simulink model "gm_Copy_of_uz_pmsm_model_9ph_21b_all_double"  (R2021b)
settings: Solver=FixedStepAuto  StartTime=0.0  StopTime=0.8  RelTol=1e-3
PreLoadFcn:
  | uz_pmsm_model_9ph_init_parameter
undefined symbols (not defined in the file or in its folder): a, b, c, friction_coefficient, inertia, k_i_d, k_i_q, k_p_d, k_p_q, Kpd, L_d, L_o1, L_o2, L_q, L_x1, L_x2, L_y1, L_y2, L_zero, polepair, psi_pm, R_1, static_friction_torque, Tnd, ts
libraries: hdlsllib x90, hdlmdlgenlib x17, slpidlib x2, simulink x2, spsAlphaBetaZerotodq0Lib x1, pid_lib x1, spsdq0toAlphaBetaZeroLib x1
(part 1 of 3)
settings Model: Creator=ts  LastModifiedBy=ts
settings SolverCC: AlgebraicLoopSolver=TrustRegion  AutoInsertRateTranBlk=on
settings DataIOCC: LimitDataPoints=on  SaveOutput=off  SaveTime=off
settings OptimizationCC: BlockReduction=off  ConditionallyExecuteInputs=off  DefaultParameterBehavior=Inlined  InheritOutputTypeSmallerThanSingle=on  LifeSpan=inf
settings DebuggingCC: AlgebraicLoopMsg=error  InheritedTsInSrcMsg=none  SingleTaskRateTransMsg=error  AllowSymbolicDim=off  StrictBusMsg=ErrorOnBusTreatedAsVector  SFUnexpectedBacktrackingDiag=warning  SFNoUnconditionalDefaultTransitionDiag=warning  SFExecutionAtInitializationDiag=none  SFMachineParentedDataDiag=warning  ArithmeticOperatorsInVariantConditions=warning
settings HardwareCC: ProdBitPerPointer=32  ProdBitPerSizeT=32  ProdBitPerPtrDiffT=32  ProdLargestAtomicFloat=None  ProdIntDivRoundTo=Undefined  ProdEndianess=Unspecified  ProdWordSize=32  ProdHWDeviceType=ASIC/FPGA->ASIC/FPGA  ProdEqTarget=off
settings SFSimCC: SimUseLocalCustomCode=off  CustomCodeUndefinedFunction=UseInterfaceOnly
settings RTWCC: RTWUseLocalCustomCode=off
settings CodeAppCC: StateflowObjectComments=on
settings GRTTargetCC: TargetLangStandard=C89/C90 (ANSI)
settings ConfigComp: CovScope=ReferencedModels  CovMetricSettings=dw  CovSaveCumulativeToWorkspaceVar=on  CovSaveSingleToWorkspaceVar=on  CovExternalEMLEnable=off  CovSFcnEnable=off

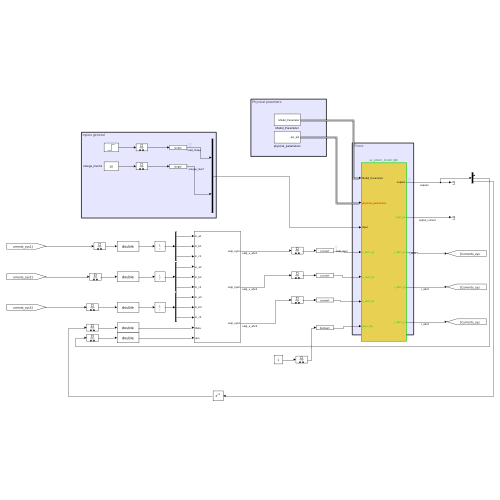
[thumbnail: Simulink's stored preview of the top-level diagram]
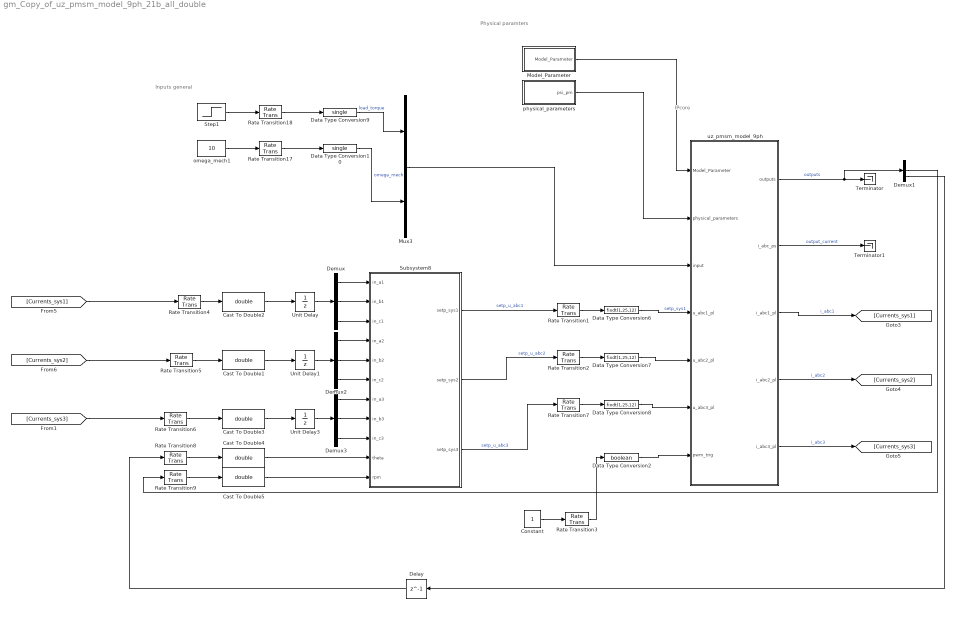
== system gm_Copy_of_uz_pmsm_model_9ph_21b_all_double ==
  note: IPcore
  note: Physical paramters
  note: Inputs general
  Cast To Double{1..5} (5 alike) : DataTypeConversion  OutDataTypeStr=double
  Constant : Constant
  Data Type Conversion10 : DataTypeConversion  OutDataTypeStr=single  RndMeth=Nearest
  Data Type Conversion2 : DataTypeConversion  OutDataTypeStr=boolean  RndMeth=Nearest
  Data Type Conversion6 : DataTypeConversion  OutDataTypeStr=fixdt(1,25,12)  RndMeth=Nearest
  Data Type Conversion7 : DataTypeConversion  OutDataTypeStr=fixdt(1,25,12)  RndMeth=Nearest
  Data Type Conversion8 : DataTypeConversion  OutDataTypeStr=fixdt(1,25,12)  RndMeth=Nearest
  Data Type Conversion9 : DataTypeConversion  OutDataTypeStr=single  RndMeth=Nearest
  Delay : Delay  DelayLength=1
  Demux{,1..3} (4 alike) : Demux  Outputs=3
  Model_Parameter : Subsystem
  Mux3 : Mux  Inputs=2
  Rate Transition{1..3,7,17..18} (6 alike) : RateTransition  OutPortSampleTime=ts
  Rate Transition{4..6,8..9} (5 alike) : RateTransition  OutPortSampleTime=1/10000
  Step1 : Step  Time=0.25  After=20  SampleTime=0
  Subsystem8 : Subsystem
  Terminator : Terminator
  Terminator1 : Terminator
  Unit Delay : UnitDelay  SampleTime=-1  HasFrameUpgradeWarning=on
  Unit Delay1 : UnitDelay  SampleTime=-1  HasFrameUpgradeWarning=on
  Unit Delay3 : UnitDelay  SampleTime=-1  HasFrameUpgradeWarning=on
  omega_mech1 : Constant  Value=10
  physical_parameters : Subsystem
  uz_pmsm_model_9ph : Subsystem  TreatAsAtomicUnit=on
  wires:
  physical_parameters/1(psi_pm) -> uz_pmsm_model_9ph/2(physical_parameters)
  uz_pmsm_model_9ph/1(outputs) -> Demux1/1, Terminator/1  "outputs"
  Model_Parameter/1(Model_Parameter) -> uz_pmsm_model_9ph/1(Model_Parameter)
  omega_mech1/1 -> Rate Transition17/1
  Rate Transition18/1 -> Data Type Conversion9/1
  Step1/1 -> Rate Transition18/1
  Data Type Conversion10/1 -> Mux3/2  "omega_mech"
  Rate Transition17/1 -> Data Type Conversion10/1
  Data Type Conversion9/1 -> Mux3/1  "load_torque"
  Mux3/1 -> uz_pmsm_model_9ph/3(input)
  uz_pmsm_model_9ph/2(i_abc_ps) -> Terminator1/1  "output_current"
  uz_pmsm_model_9ph/3(i_abc1_pl) -> [Currents_sys1]  "i_abc1"
  uz_pmsm_model_9ph/5(i_abc3_pl) -> [Currents_sys3]  "i_abc3"
  uz_pmsm_model_9ph/4(i_abc2_pl) -> [Currents_sys2]  "i_abc2"
  Subsystem8/1(setp_sys1) -> Rate Transition1/1  "setp_u_abc1"
  Data Type Conversion6/1 -> uz_pmsm_model_9ph/4(u_abc1_pl)  "setp_sys1"
  Subsystem8/2(setp_sys2) -> Rate Transition2/1  "setp_u_abc2"
  Subsystem8/3(setp_sys3) -> Rate Transition7/1  "setp_u_abc3"
  Data Type Conversion8/1 -> uz_pmsm_model_9ph/6(u_abc3_pl)
  Data Type Conversion7/1 -> uz_pmsm_model_9ph/5(u_abc2_pl)
  Unit Delay3/1 -> Demux3/1
  Demux/2 -> Subsystem8/2(in_b1)
  Demux2/1 -> Subsystem8/4(in_a2)
  Demux3/2 -> Subsystem8/8(in_b3)
  Unit Delay1/1 -> Demux2/1
  Demux/3 -> Subsystem8/3(in_c1)
  [Currents_sys1] -> Rate Transition4/1
  [Currents_sys2] -> Rate Transition5/1
  Demux3/3 -> Subsystem8/9(in_c3)
  Unit Delay/1 -> Demux/1
  [Currents_sys3] -> Rate Transition6/1
  Demux3/1 -> Subsystem8/7(in_a3)
  Demux/1 -> Subsystem8/1(in_a1)
  Demux2/2 -> Subsystem8/5(in_b2)
  Demux2/3 -> Subsystem8/6(in_c2)
  Cast To Double1/1 -> Unit Delay1/1
  Cast To Double2/1 -> Unit Delay/1
  Cast To Double3/1 -> Unit Delay3/1
  Rate Transition1/1 -> Data Type Conversion6/1
  Rate Transition2/1 -> Data Type Conversion7/1
  Rate Transition7/1 -> Data Type Conversion8/1
  Data Type Conversion2/1 -> uz_pmsm_model_9ph/7(pwm_trig)
  Constant/1 -> Rate Transition3/1
  Rate Transition3/1 -> Data Type Conversion2/1
  Demux1/3 -> Delay/1
  Demux1/2 -> Rate Transition9/1
  Cast To Double4/1 -> Subsystem8/10(theta)
  Cast To Double5/1 -> Subsystem8/11(rpm)
  Delay/1 -> Rate Transition8/1
  Rate Transition4/1 -> Cast To Double2/1
  Rate Transition5/1 -> Cast To Double1/1
  Rate Transition6/1 -> Cast To Double3/1
  Rate Transition8/1 -> Cast To Double4/1
  Rate Transition9/1 -> Cast To Double5/1

== system gm_Copy_of_uz_pmsm_model_9ph_21b_all_double/Model_Parameter ==
  note: This flag determines if omega_mech is used as an input value or
      | if the mechanical system is simulated by the model
  Bus Creator : BusCreator  Inputs=4
  Constant3 : Constant  Value=0
  Data Type Conversion{3..4,9..10} (4 alike) : DataTypeConversion  OutDataTypeStr=boolean
  Rate Transition{6,8,17..18} (4 alike) : RateTransition  OutPortSampleTime=ts
  simulate_mechanical : Constant  Value=false
  simulate_mechanical1 : Constant  Value=false
  simulate_mechanical2 : Constant  Value=false
  Model_Parameter : Outport
  wires:
  simulate_mechanical2/1 -> Rate Transition18/1
  simulate_mechanical/1 -> Rate Transition8/1
  Rate Transition8/1 -> Data Type Conversion4/1
  Rate Transition6/1 -> Data Type Conversion3/1
  Constant3/1 -> Rate Transition6/1
  simulate_mechanical1/1 -> Rate Transition17/1
  Rate Transition17/1 -> Data Type Conversion9/1
  Rate Transition18/1 -> Data Type Conversion10/1
  Data Type Conversion10/1 -> Bus Creator/4  "control_dq_abc"
  Data Type Conversion9/1 -> Bus Creator/3  "switch_pspl"
  Data Type Conversion4/1 -> Bus Creator/2  "simulate_mechanical"
  Bus Creator/1 -> Model_Parameter/1
  Data Type Conversion3/1 -> Bus Creator/1  "reset_integrators"

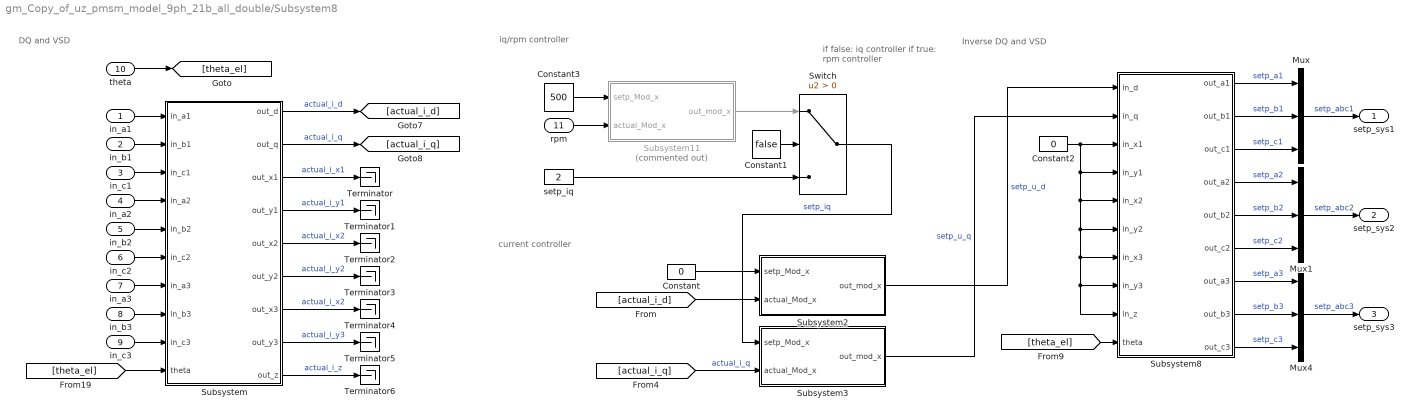
== system gm_Copy_of_uz_pmsm_model_9ph_21b_all_double/Subsystem8 ==
  note: DQ and VSD
  note: current controller
  note: iq/rpm controller
  note: if false: iq controller
      | if true: rpm controller
  note: Inverse DQ and VSD
  in_a1 : Inport
  in_b1 : Inport  Port=2
  in_c1 : Inport  Port=3
  in_a2 : Inport  Port=4
  in_b2 : Inport  Port=5
  in_c2 : Inport  Port=6
  in_a3 : Inport  Port=7
  in_b3 : Inport  Port=8
  in_c3 : Inport  Port=9
  theta : Inport  Port=10
  rpm : Inport  Port=11
  Constant : Constant  Value=0
  Constant1 : Constant  Value=false
  Constant2 : Constant  Value=0
  Constant3 : Constant  Value=500
  Mux : Mux  Inputs=3
  Mux1 : Mux  Inputs=3
  Mux4 : Mux  Inputs=3
  Subsystem : Subsystem
  Subsystem11 : Subsystem  Commented=on
  Subsystem2 : Subsystem
  Subsystem3 : Subsystem
  Subsystem8 : Subsystem
  Switch : Switch  Criteria=u2 > Threshold
  Terminator{,1..6} (7 alike) : Terminator
  setp_iq : Constant  Value=2
  setp_sys1 : Outport
  setp_sys2 : Outport  Port=2
  setp_sys3 : Outport  Port=3
  wires:
  Subsystem/4(out_y1) -> Terminator1/1  "actual_i_y1"
  Subsystem8/1(out_a1) -> Mux/1  "setp_a1"
  in_b1/1 -> Subsystem/2(in_b1)
  [theta_el] -> Subsystem8/10(theta)
  Subsystem8/2(out_b1) -> Mux/2  "setp_b1"
  Subsystem8/3(out_c1) -> Mux/3  "setp_c1"
  Subsystem/3(out_x1) -> Terminator/1  "actual_i_x1"
  in_c1/1 -> Subsystem/3(in_c1)
  [actual_i_d] -> Subsystem2/2(actual_Mod_x)
  Constant/1 -> Subsystem2/1(setp_Mod_x)
  Subsystem/6(out_y2) -> Terminator3/1  "actual_i_y2"
  Subsystem/5(out_x2) -> Terminator2/1  "actual_i_x2"
  in_a1/1 -> Subsystem/1(in_a1)
  [actual_i_q] -> Subsystem3/2(actual_Mod_x)  "actual_i_q"
  in_b2/1 -> Subsystem/5(in_b2)
  in_a2/1 -> Subsystem/4(in_a2)
  in_c2/1 -> Subsystem/6(in_c2)
  theta/1 -> [theta_el]
  Mux/1 -> setp_sys1/1  "setp_abc1"
  Subsystem/8(out_y3) -> Terminator5/1  "actual_i_y3"
  Subsystem/7(out_x3) -> Terminator4/1  "actual_i_x2"
  Subsystem/9(out_z) -> Terminator6/1  "actual_i_z"
  in_c3/1 -> Subsystem/9(in_c3)
  in_b3/1 -> Subsystem/8(in_b3)
  in_a3/1 -> Subsystem/7(in_a3)
  Mux1/1 -> setp_sys2/1  "setp_abc2"
  Subsystem8/6(out_c2) -> Mux1/3  "setp_c2"
  Subsystem8/5(out_b2) -> Mux1/2  "setp_b2"
  Subsystem8/4(out_a2) -> Mux1/1  "setp_a2"
  Mux4/1 -> setp_sys3/1  "setp_abc3"
  Subsystem8/7(out_a3) -> Mux4/1  "setp_a3"
  Subsystem8/8(out_b3) -> Mux4/2  "setp_b3"
  Subsystem8/9(out_c3) -> Mux4/3  "setp_c3"
  rpm/1 -> Subsystem11/2(actual_Mod_x)
  Subsystem/1(out_d) -> [actual_i_d]  "actual_i_d"
  Subsystem/2(out_q) -> [actual_i_q]  "actual_i_q"
  [theta_el] -> Subsystem/10(theta)
  Constant2/1 -> Subsystem8/3(in_x1), Subsystem8/8(in_y3), Subsystem8/9(in_z), Subsystem8/7(in_x3), Subsystem8/6(in_y2), Subsystem8/5(in_x2), Subsystem8/4(in_y1)
  Subsystem11/1(out_mod_x) -> Switch/1
  Switch/1 -> Subsystem3/1(setp_Mod_x)  "setp_iq"
  Constant1/1 -> Switch/2
  setp_iq/1 -> Switch/3
  Constant3/1 -> Subsystem11/1(setp_Mod_x)
  Subsystem3/1(out_mod_x) -> Subsystem8/2(in_q)  "setp_u_q"
  Subsystem2/1(out_mod_x) -> Subsystem8/1(in_d)  "setp_u_d"

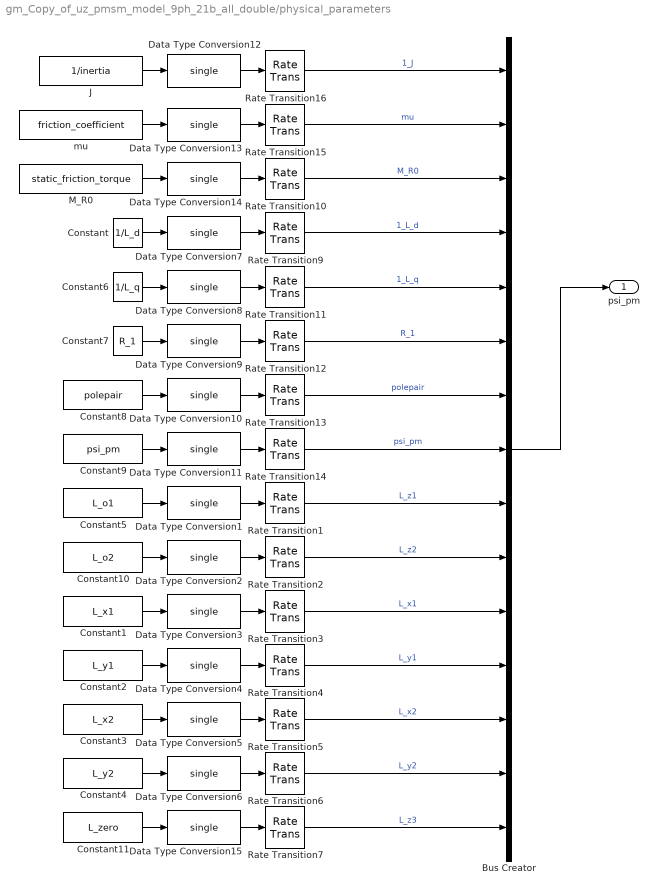
== system gm_Copy_of_uz_pmsm_model_9ph_21b_all_double/physical_parameters ==
  Bus Creator : BusCreator  Inputs=15
  Constant : Constant  Value=1/L_d
  Constant1 : Constant  Value=L_x1
  Constant10 : Constant  Value=L_o2
  Constant11 : Constant  Value=L_zero
  Constant2 : Constant  Value=L_y1
  Constant3 : Constant  Value=L_x2
  Constant4 : Constant  Value=L_y2
  Constant5 : Constant  Value=L_o1
  Constant6 : Constant  Value=1/L_q
  Constant7 : Constant  Value=R_1
  Constant8 : Constant  Value=polepair
  Constant9 : Constant  Value=psi_pm
  Data Type Conversion{1..15} (15 alike) : DataTypeConversion  OutDataTypeStr=single
  J : Constant  Value=1/inertia
  M_R0 : Constant  Value=static_friction_torque
  Rate Transition{1..7,9..16} (15 alike) : RateTransition  OutPortSampleTime=ts
  mu : Constant  Value=friction_coefficient
  psi_pm : Outport
  wires:
  Data Type Conversion12/1 -> Rate Transition16/1
  Data Type Conversion7/1 -> Rate Transition9/1
  Rate Transition10/1 -> Bus Creator/3  "M_R0"
  Rate Transition14/1 -> Bus Creator/8  "psi_pm"
  Data Type Conversion14/1 -> Rate Transition10/1
  Rate Transition12/1 -> Bus Creator/6  "R_1"
  Rate Transition16/1 -> Bus Creator/1  "1_J"
  Rate Transition13/1 -> Bus Creator/7  "polepair"
  Bus Creator/1 -> psi_pm/1
  Data Type Conversion11/1 -> Rate Transition14/1
  Constant8/1 -> Data Type Conversion10/1
  Data Type Conversion9/1 -> Rate Transition12/1
  Rate Transition15/1 -> Bus Creator/2  "mu"
  Constant6/1 -> Data Type Conversion8/1
  Rate Transition9/1 -> Bus Creator/4  "1_L_d"
  J/1 -> Data Type Conversion12/1
  Data Type Conversion8/1 -> Rate Transition11/1
  Data Type Conversion10/1 -> Rate Transition13/1
  mu/1 -> Data Type Conversion13/1
  M_R0/1 -> Data Type Conversion14/1
  Rate Transition11/1 -> Bus Creator/5  "1_L_q"
  Data Type Conversion13/1 -> Rate Transition15/1
  Constant7/1 -> Data Type Conversion9/1
  Constant9/1 -> Data Type Conversion11/1
  Constant/1 -> Data Type Conversion7/1
  Data Type Conversion1/1 -> Rate Transition1/1
  Data Type Conversion2/1 -> Rate Transition2/1
  Data Type Conversion3/1 -> Rate Transition3/1
  Data Type Conversion4/1 -> Rate Transition4/1
  Data Type Conversion5/1 -> Rate Transition5/1
  Data Type Conversion6/1 -> Rate Transition6/1
  Constant11/1 -> Data Type Conversion15/1
  Data Type Conversion15/1 -> Rate Transition7/1
  Rate Transition1/1 -> Bus Creator/9  "L_z1"
  Rate Transition7/1 -> Bus Creator/15  "L_z3"
  Rate Transition6/1 -> Bus Creator/14  "L_y2"
  Rate Transition5/1 -> Bus Creator/13  "L_x2"
  Rate Transition4/1 -> Bus Creator/12  "L_y1"
  Rate Transition3/1 -> Bus Creator/11  "L_x1"
  Rate Transition2/1 -> Bus Creator/10  "L_z2"
  Constant4/1 -> Data Type Conversion6/1
  Constant3/1 -> Data Type Conversion5/1
  Constant2/1 -> Data Type Conversion4/1
  Constant1/1 -> Data Type Conversion3/1
  Constant5/1 -> Data Type Conversion1/1
  Constant10/1 -> Data Type Conversion2/1

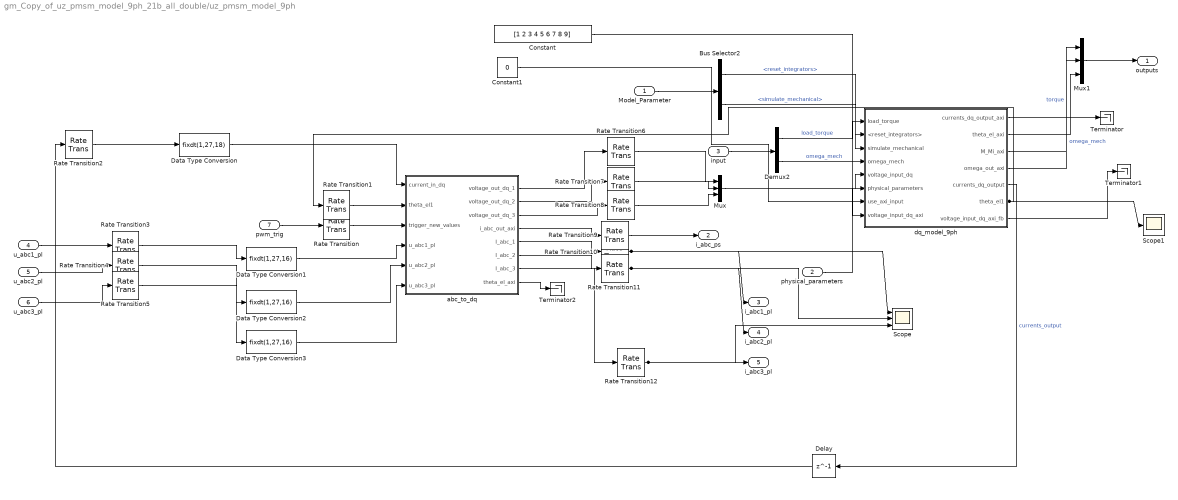
== system gm_Copy_of_uz_pmsm_model_9ph_21b_all_double/uz_pmsm_model_9ph ==
  Model_Parameter : Inport
  physical_parameters : Inport  Port=2
  input : Inport  Port=3
  u_abc1_pl : Inport  Port=4
  u_abc2_pl : Inport  Port=5
  u_abc3_pl : Inport  Port=6
  pwm_trig : Inport  Port=7
  Bus Selector2 : BusSelector  OutputSignals=reset_integrators,simulate_mechanical
  Constant : Constant  Value=[1 2 3 4 5 6 7 8 9]  OutDataTypeStr=single  SampleTime=-1
  Constant1 : Constant  Value=0  OutDataTypeStr=boolean  SampleTime=ts
  Data Type Conversion : DataTypeConversion  OutDataTypeStr=fixdt(1,27,18)
  Data Type Conversion1 : DataTypeConversion  OutDataTypeStr=fixdt(1,27,16)
  Data Type Conversion2 : DataTypeConversion  OutDataTypeStr=fixdt(1,27,16)
  Data Type Conversion3 : DataTypeConversion  OutDataTypeStr=fixdt(1,27,16)
  Delay : Delay  DelayLength=1
  Demux2 : Demux  Outputs=2
  Mux : Mux  Inputs=3
  Mux1 : Mux  Inputs=3
  Rate Transition{,1..5} (6 alike) : RateTransition  OutPortSampleTime=1/100e6
  Rate Transition{6..12} (7 alike) : RateTransition
  Scope : Scope  NumInputPorts=3
  Scope1 : Scope  NumInputPorts=3
  Terminator : Terminator
  Terminator1 : Terminator
  Terminator2 : Terminator
  abc_to_dq : Subsystem  TreatAsAtomicUnit=on
  dq_model_9ph : Subsystem  TreatAsAtomicUnit=on
  outputs : Outport
  i_abc_ps : Outport  Port=2
  i_abc1_pl : Outport  Port=3
  i_abc2_pl : Outport  Port=4
  i_abc3_pl : Outport  Port=5
  wires:
  Rate Transition5/1 -> Data Type Conversion3/1
  Data Type Conversion3/1 -> abc_to_dq/6(u_abc3_pl)
  Data Type Conversion1/1 -> abc_to_dq/4(u_abc1_pl)
  Rate Transition3/1 -> Data Type Conversion1/1
  Rate Transition4/1 -> Data Type Conversion2/1
  Data Type Conversion2/1 -> abc_to_dq/5(u_abc2_pl)
  dq_model_9ph/5(currents_dq_output) -> Delay/1  "currents_output"
  Data Type Conversion/1 -> abc_to_dq/1(current_in_dq)
  abc_to_dq/8(theta_el_axi) -> Terminator2/1
  Rate Transition12/1 -> i_abc3_pl/1, Scope/3
  Rate Transition11/1 -> i_abc2_pl/1, Scope/2
  Rate Transition10/1 -> i_abc1_pl/1, Scope/1
  Rate Transition9/1 -> i_abc_ps/1
  Rate Transition8/1 -> Mux/3
  Rate Transition7/1 -> Mux/2
  Rate Transition6/1 -> Mux/1
  Rate Transition2/1 -> Data Type Conversion/1
  Rate Transition1/1 -> abc_to_dq/2(theta_el1)
  Rate Transition/1 -> abc_to_dq/3(trigger_new_values)
  dq_model_9ph/7(voltage_input_dq_axi_fb) -> Terminator1/1
  Constant1/1 -> dq_model_9ph/7(use_axi_input)
  Constant/1 -> dq_model_9ph/8(voltage_input_dq_axi)
  dq_model_9ph/1(currents_dq_output_axi) -> Terminator/1
  dq_model_9ph/2(theta_el_axi) -> Mux1/3
  abc_to_dq/3(voltage_out_dq_3) -> Rate Transition8/1
  abc_to_dq/2(voltage_out_dq_2) -> Rate Transition7/1
  abc_to_dq/1(voltage_out_dq_1) -> Rate Transition6/1
  Mux/1 -> dq_model_9ph/5(voltage_input_dq)
  dq_model_9ph/6(theta_el1) -> Scope1/2, Rate Transition1/1
  Delay/1 -> Rate Transition2/1
  abc_to_dq/7(I_abc_3) -> Rate Transition12/1
  abc_to_dq/6(I_abc_2) -> Rate Transition11/1
  abc_to_dq/5(I_abc_1) -> Rate Transition10/1
  abc_to_dq/4(i_abc_out_axi) -> Rate Transition9/1
  u_abc3_pl/1 -> Rate Transition5/1
  u_abc2_pl/1 -> Rate Transition4/1
  u_abc1_pl/1 -> Rate Transition3/1
  pwm_trig/1 -> Rate Transition/1
  Mux1/1 -> outputs/1
  Bus Selector2/2 -> dq_model_9ph/3(simulate_mechanical)  "<simulate_mechanical>"
  Bus Selector2/1 -> dq_model_9ph/2(<reset_integrators>)  "<reset_integrators>"
  Model_Parameter/1 -> Bus Selector2/1
  input/1 -> Demux2/1
  Demux2/2 -> dq_model_9ph/4(omega_mech)  "omega_mech"
  Demux2/1 -> dq_model_9ph/1(load_torque)  "load_torque"
  dq_model_9ph/3(M_Mi_axi) -> Mux1/1  "torque"
  dq_model_9ph/4(omega_out_axi) -> Mux1/2  "omega_mech"
  physical_parameters/1 -> dq_model_9ph/6(physical_parameters)

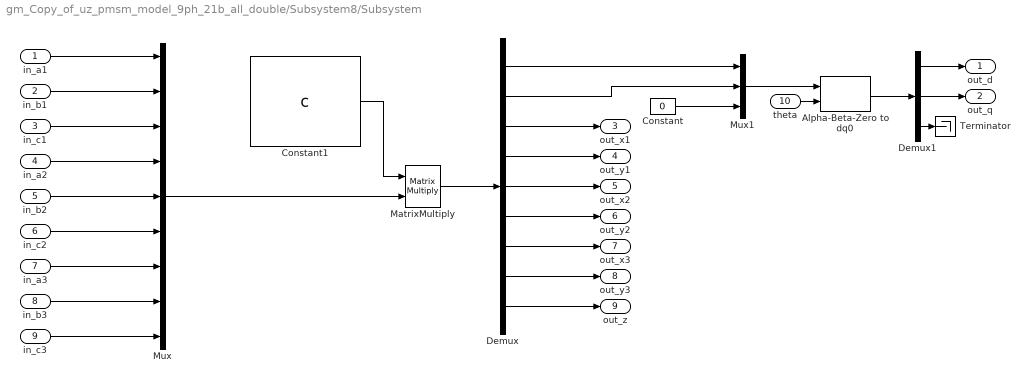
== system gm_Copy_of_uz_pmsm_model_9ph_21b_all_double/Subsystem8/Subsystem ==
  in_a1 : Inport
  in_b1 : Inport  Port=2
  in_c1 : Inport  Port=3
  in_a2 : Inport  Port=4
  in_b2 : Inport  Port=5
  in_c2 : Inport  Port=6
  in_a3 : Inport  Port=7
  in_b3 : Inport  Port=8
  in_c3 : Inport  Port=9
  theta : Inport  Port=10
  Alpha-Beta-Zero to dq0 : spsAlphaBetaZerotodq0Lib/Alpha-Beta-Zero to dq0  Alignment=90 degrees behind phase A axis
      settings: SourceProductBaseCode=PS
  Constant : Constant  Value=0
  Constant1 : Constant  Value=c
  Demux : Demux  Outputs=9
  Demux1 : Demux  Outputs=3
  MatrixMultiply : Product  Multiplication=Matrix(*)
  Mux : Mux  Inputs=9
  Mux1 : Mux  Inputs=3
  Terminator : Terminator
  out_d : Outport
  out_q : Outport  Port=2
  out_x1 : Outport  Port=3
  out_y1 : Outport  Port=4
  out_x2 : Outport  Port=5
  out_y2 : Outport  Port=6
  out_x3 : Outport  Port=7
  out_y3 : Outport  Port=8
  out_z : Outport  Port=9
  wires:
  Demux/6 -> out_y2/1
  Demux/4 -> out_y1/1
  in_a1/1 -> Mux/1
  Demux/5 -> out_x2/1
  MatrixMultiply/1 -> Demux/1
  Demux/3 -> out_x1/1
  in_c3/1 -> Mux/9
  Demux/7 -> out_x3/1
  Demux/8 -> out_y3/1
  Demux/9 -> out_z/1
  theta/1 -> Alpha-Beta-Zero to dq0/2
  Demux1/3 -> Terminator/1
  Demux/1 -> Mux1/1
  Mux1/1 -> Alpha-Beta-Zero to dq0/1
  Demux/2 -> Mux1/2
  Demux1/1 -> out_d/1
  Demux1/2 -> out_q/1
  Constant/1 -> Mux1/3
  Alpha-Beta-Zero to dq0/1 -> Demux1/1
  Constant1/1 -> MatrixMultiply/1
  Mux/1 -> MatrixMultiply/2
  in_b1/1 -> Mux/2
  in_c1/1 -> Mux/3
  in_a2/1 -> Mux/4
  in_b2/1 -> Mux/5
  in_c2/1 -> Mux/6
  in_a3/1 -> Mux/7
  in_b3/1 -> Mux/8

== system gm_Copy_of_uz_pmsm_model_9ph_21b_all_double/Subsystem8/Subsystem11 ==
  setp_Mod_x : Inport
  actual_Mod_x : Inport  Port=2
  Add : Sum  Inputs=+-
  Data Type Conversion8 : DataTypeConversion  OutDataTypeStr=double
  PID Controller2 : pid_lib/PID Controller  Controller=PI  Form=Ideal  TimeDomain=Continuous-time  UseExternalTs=off  SampleTime=-1  IntegratorMethod=Forward Euler  FilterMethod=Forward Euler  ControllerParametersSource=internal  P=Kpd  I=1/Tnd  D=0  N=100  UseFilter=on  TunerSelectOption=Transfer Function Based (PID Tuner App)  InitialConditionSource=internal  InitialConditionForIntegrator=0  InitialConditionForFilter=0  DifferentiatorICPrevScaledInput=0  ExternalReset=none  TrackingMode=off  Kt=1  LimitOutput=on  SatLimitsSource=internal  UpperSaturationLimit=50  LowerSaturationLimit=-50  LinearizeAsGain=on  AntiWindupMode=clamping  Kb=1  POutMin=[]  POutMax=[]  IOutMin=[]  IOutMax=[]  DOutMin=[]  DOutMax=[]  NOutMin=[]  NOutMax=[]  SumOutMin=[]  SumOutMax=[]  SaturationOutMin=[]  SaturationOutMax=[]  PParamMin=[]  PParamMax=[]  IParamMin=[]  IParamMax=[]  DParamMin=[]  DParamMax=[]  NParamMin=[]  NParamMax=[]  KbParamMin=[]  KbParamMax=[]  KtParamMin=[]  KtParamMax=[]  KbOutMin=[]  KbOutMax=[]  KtOutMin=[]  KtOutMax=[]  IntegratorOutMin=[]  IntegratorOutMax=[]  FilterOutMin=[]  FilterOutMax=[]  SumI1OutMin=[]  SumI1OutMax=[]  SumI2OutMin=[]  SumI2OutMax=[]  SumI3OutMin=[]  SumI3OutMax=[]  SumI4OutMin=[]  SumI4OutMax=[]  SumDOutMin=[]  SumDOutMax=[]  DifferentiatorOutMin=[]  DifferentiatorOutMax=[]  FilterDiffOutCoefMin=[]  FilterDiffOutCoefMax=[]  ReciprocalOutMin=[]  ReciprocalOutMax=[]  SumDenOutMin=[]  SumDenOutMax=[]  SumNumOutMin=[]  SumNumOutMax=[]  DivideOutMin=[]  DivideOutMax=[]  UdiffTsProdOutMin=[]  UdiffTsProdOutMax=[]  NTsProdOutMin=[]  NTsProdOutMax=[]  UintegralTsProdOutMin=[]  UintegralTsProdOutMax=[]  UngainTsProdOutMin=[]  UngainTsProdOutMax=[]  IntegratorContinuousStateAttributes=''  IntegratorStateMustResolveToSignalObject=off  IntegratorRTWStateStorageClass=Auto  FilterContinuousStateAttributes=''  FilterStateMustResolveToSignalObject=off  FilterRTWStateStorageClass=Auto  ParallelPVariant=Passthrough  IdealPVariant=InternalParameters  IVariant=InternalParameters  DVariant=Disabled  IntegratorVariant=Continuous  SatVariant=Enabled  AWVariant=ContClampingIdeal  PCopyVariant=InternalParamsIdeal  TRVariant=Disabled  FdbkBlocksVariant=Forward  IdealPFdbkVariant=Disabled  SatFdbkVariant=Disabled  DerivativeFilterVariant=Disabled  NVariant=Disabled  NCopyVariant=Disabled_SignalSpec  FilterICVariant=Disabled  IntegratorICVariant=InternalICs  ExternalResetVariant=Disabled  TRSumVariant=Passthrough  SumFdbkVariant=Disabled  SumVariant=Sum_PI  TsampFilterVariant=InternalTs  TsampNgainVariant=Passthrough  TsampIntegralVariant=Passthrough  ExternalSaturationOutDataTypeStr=Inherit: Same as second input
  out_mod_x : Outport
  wires:
  Add/1 -> Data Type Conversion8/1
  actual_Mod_x/1 -> Add/2
  Data Type Conversion8/1 -> PID Controller2/1
  setp_Mod_x/1 -> Add/1
  PID Controller2/1 -> out_mod_x/1

== system gm_Copy_of_uz_pmsm_model_9ph_21b_all_double/Subsystem8/Subsystem2 ==
  setp_Mod_x : Inport
  actual_Mod_x : Inport  Port=2
  Add : Sum  Inputs=+-
  Data Type Conversion8 : DataTypeConversion  OutDataTypeStr=double
  PID Controller2 : slpidlib/PID Controller  Controller=PI  Form=Ideal  TimeDomain=Continuous-time  UseExternalTs=off  SampleTime=-1  IntegratorMethod=Forward Euler  FilterMethod=Forward Euler  ControllerParametersSource=internal  P=k_p_d  I=k_i_d  D=0  UseFilter=on  N=100  TunerSelectOption=Transfer Function Based (PID Tuner App)  InitialConditionSource=internal  InitialConditionForIntegrator=0  InitialConditionForFilter=0  DifferentiatorICPrevScaledInput=0  ExternalReset=none  TrackingMode=off  Kt=1  LimitOutput=on  SatLimitsSource=internal  UpperSaturationLimit=100  LowerSaturationLimit=-100  LinearizeAsGain=on  AntiWindupMode=clamping  Kb=1  POutMin=[]  POutMax=[]  IOutMin=[]  IOutMax=[]  DOutMin=[]  DOutMax=[]  NOutMin=[]  NOutMax=[]  SumOutMin=[]  SumOutMax=[]  SaturationOutMin=[]  SaturationOutMax=[]  PParamMin=[]  PParamMax=[]  IParamMin=[]  IParamMax=[]  DParamMin=[]  DParamMax=[]  NParamMin=[]  NParamMax=[]  KbParamMin=[]  KbParamMax=[]  KtParamMin=[]  KtParamMax=[]  KbOutMin=[]  KbOutMax=[]  KtOutMin=[]  KtOutMax=[]  IntegratorOutMin=[]  IntegratorOutMax=[]  FilterOutMin=[]  FilterOutMax=[]  SumI1OutMin=[]  SumI1OutMax=[]  SumI2OutMin=[]  SumI2OutMax=[]  SumI3OutMin=[]  SumI3OutMax=[]  SumI4OutMin=[]  SumI4OutMax=[]  SumDOutMin=[]  SumDOutMax=[]  DifferentiatorOutMin=[]  DifferentiatorOutMax=[]  FilterDiffOutCoefMin=[]  FilterDiffOutCoefMax=[]  ReciprocalOutMin=[]  ReciprocalOutMax=[]  SumDenOutMin=[]  SumDenOutMax=[]  SumNumOutMin=[]  SumNumOutMax=[]  DivideOutMin=[]  DivideOutMax=[]  UdiffTsProdOutMin=[]  UdiffTsProdOutMax=[]  NTsProdOutMin=[]  NTsProdOutMax=[]  UintegralTsProdOutMin=[]  UintegralTsProdOutMax=[]  UngainTsProdOutMin=[]  UngainTsProdOutMax=[]  IntegratorContinuousStateAttributes=''  IntegratorStateMustResolveToSignalObject=off  IntegratorRTWStateStorageClass=Auto  FilterContinuousStateAttributes=''  FilterStateMustResolveToSignalObject=off  FilterRTWStateStorageClass=Auto  ParallelPVariant=Passthrough  IdealPVariant=InternalParameters  IVariant=InternalParameters  DVariant=Disabled  IntegratorVariant=Continuous  SatVariant=Enabled  AWVariant=ContClampingIdeal  PCopyVariant=InternalParamsIdeal  TRVariant=Disabled  FdbkBlocksVariant=Forward  IdealPFdbkVariant=Disabled  SatFdbkVariant=Disabled  DerivativeFilterVariant=Disabled  NVariant=Disabled  NCopyVariant=Disabled_SignalSpec  FilterICVariant=Disabled  IntegratorICVariant=InternalICs  ExternalResetVariant=Disabled  TRSumVariant=Passthrough  SumFdbkVariant=Disabled  SumVariant=Sum_PI  TsampFilterVariant=InternalTs  TsampNgainVariant=Passthrough  TsampIntegralVariant=Passthrough  ExternalSaturationOutDataTypeStr=Inherit: Same as second input
  out_mod_x : Outport
  wires:
  Add/1 -> Data Type Conversion8/1
  actual_Mod_x/1 -> Add/2
  Data Type Conversion8/1 -> PID Controller2/1
  setp_Mod_x/1 -> Add/1
  PID Controller2/1 -> out_mod_x/1

== system gm_Copy_of_uz_pmsm_model_9ph_21b_all_double/Subsystem8/Subsystem3 ==
  setp_Mod_x : Inport
  actual_Mod_x : Inport  Port=2
  Add : Sum  Inputs=+-
  Data Type Conversion8 : DataTypeConversion  OutDataTypeStr=double
  PID Controller2 : slpidlib/PID Controller  Controller=PI  Form=Ideal  TimeDomain=Continuous-time  UseExternalTs=off  SampleTime=-1  IntegratorMethod=Forward Euler  FilterMethod=Forward Euler  ControllerParametersSource=internal  P=k_p_q  I=k_i_q  D=0  UseFilter=on  N=100  TunerSelectOption=Transfer Function Based (PID Tuner App)  InitialConditionSource=internal  InitialConditionForIntegrator=0  InitialConditionForFilter=0  DifferentiatorICPrevScaledInput=0  ExternalReset=none  TrackingMode=off  Kt=1  LimitOutput=on  SatLimitsSource=internal  UpperSaturationLimit=100  LowerSaturationLimit=-100  LinearizeAsGain=on  AntiWindupMode=clamping  Kb=1  POutMin=[]  POutMax=[]  IOutMin=[]  IOutMax=[]  DOutMin=[]  DOutMax=[]  NOutMin=[]  NOutMax=[]  SumOutMin=[]  SumOutMax=[]  SaturationOutMin=[]  SaturationOutMax=[]  PParamMin=[]  PParamMax=[]  IParamMin=[]  IParamMax=[]  DParamMin=[]  DParamMax=[]  NParamMin=[]  NParamMax=[]  KbParamMin=[]  KbParamMax=[]  KtParamMin=[]  KtParamMax=[]  KbOutMin=[]  KbOutMax=[]  KtOutMin=[]  KtOutMax=[]  IntegratorOutMin=[]  IntegratorOutMax=[]  FilterOutMin=[]  FilterOutMax=[]  SumI1OutMin=[]  SumI1OutMax=[]  SumI2OutMin=[]  SumI2OutMax=[]  SumI3OutMin=[]  SumI3OutMax=[]  SumI4OutMin=[]  SumI4OutMax=[]  SumDOutMin=[]  SumDOutMax=[]  DifferentiatorOutMin=[]  DifferentiatorOutMax=[]  FilterDiffOutCoefMin=[]  FilterDiffOutCoefMax=[]  ReciprocalOutMin=[]  ReciprocalOutMax=[]  SumDenOutMin=[]  SumDenOutMax=[]  SumNumOutMin=[]  SumNumOutMax=[]  DivideOutMin=[]  DivideOutMax=[]  UdiffTsProdOutMin=[]  UdiffTsProdOutMax=[]  NTsProdOutMin=[]  NTsProdOutMax=[]  UintegralTsProdOutMin=[]  UintegralTsProdOutMax=[]  UngainTsProdOutMin=[]  UngainTsProdOutMax=[]  IntegratorContinuousStateAttributes=''  IntegratorStateMustResolveToSignalObject=off  IntegratorRTWStateStorageClass=Auto  FilterContinuousStateAttributes=''  FilterStateMustResolveToSignalObject=off  FilterRTWStateStorageClass=Auto  ParallelPVariant=Passthrough  IdealPVariant=InternalParameters  IVariant=InternalParameters  DVariant=Disabled  IntegratorVariant=Continuous  SatVariant=Enabled  AWVariant=ContClampingIdeal  PCopyVariant=InternalParamsIdeal  TRVariant=Disabled  FdbkBlocksVariant=Forward  IdealPFdbkVariant=Disabled  SatFdbkVariant=Disabled  DerivativeFilterVariant=Disabled  NVariant=Disabled  NCopyVariant=Disabled_SignalSpec  FilterICVariant=Disabled  IntegratorICVariant=InternalICs  ExternalResetVariant=Disabled  TRSumVariant=Passthrough  SumFdbkVariant=Disabled  SumVariant=Sum_PI  TsampFilterVariant=InternalTs  TsampNgainVariant=Passthrough  TsampIntegralVariant=Passthrough  ExternalSaturationOutDataTypeStr=Inherit: Same as second input
  out_mod_x : Outport
  wires:
  PID Controller2/1 -> out_mod_x/1
  setp_Mod_x/1 -> Add/1
  Data Type Conversion8/1 -> PID Controller2/1
  actual_Mod_x/1 -> Add/2
  Add/1 -> Data Type Conversion8/1

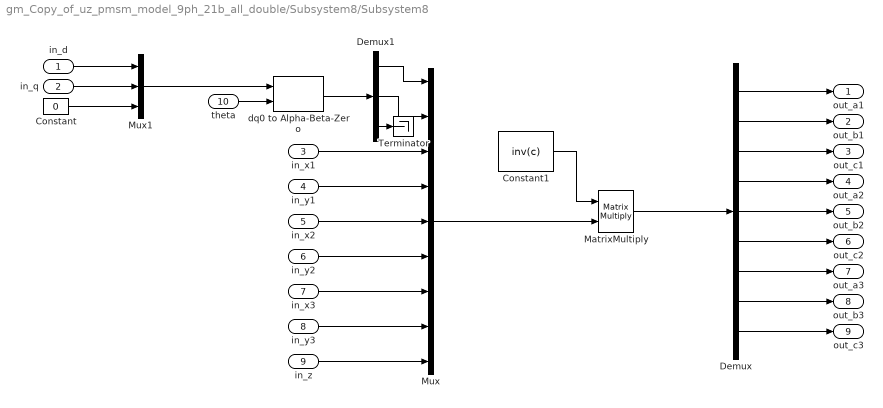
== system gm_Copy_of_uz_pmsm_model_9ph_21b_all_double/Subsystem8/Subsystem8 ==
  in_d : Inport
  in_q : Inport  Port=2
  in_x1 : Inport  Port=3
  in_y1 : Inport  Port=4
  in_x2 : Inport  Port=5
  in_y2 : Inport  Port=6
  in_x3 : Inport  Port=7
  in_y3 : Inport  Port=8
  in_z : Inport  Port=9
  theta : Inport  Port=10
  Constant : Constant  Value=0
  Constant1 : Constant  Value=inv(c)
  Demux : Demux  Outputs=9
  Demux1 : Demux  Outputs=3
  MatrixMultiply : Product  Multiplication=Matrix(*)
  Mux : Mux  Inputs=9
  Mux1 : Mux  Inputs=3
  Terminator : Terminator
  dq0 to Alpha-Beta-Zero : spsdq0toAlphaBetaZeroLib/dq0 to Alpha-Beta-Zero  Alignment=90 degrees behind phase A axis
      settings: SourceProductBaseCode=PS
  out_a1 : Outport
  out_b1 : Outport  Port=2
  out_c1 : Outport  Port=3
  out_a2 : Outport  Port=4
  out_b2 : Outport  Port=5
  out_c2 : Outport  Port=6
  out_a3 : Outport  Port=7
  out_b3 : Outport  Port=8
  out_c3 : Outport  Port=9
  wires:
  in_x3/1 -> Mux/7
  in_y3/1 -> Mux/8
  MatrixMultiply/1 -> Demux/1
  in_y2/1 -> Mux/6
  Demux/1 -> out_a1/1
  in_x1/1 -> Mux/3
  in_y1/1 -> Mux/4
  Mux/1 -> MatrixMultiply/2
  in_x2/1 -> Mux/5
  in_z/1 -> Mux/9
  Constant/1 -> Mux1/3
  in_q/1 -> Mux1/2
  in_d/1 -> Mux1/1
  Mux1/1 -> dq0 to Alpha-Beta-Zero/1
  theta/1 -> dq0 to Alpha-Beta-Zero/2
  dq0 to Alpha-Beta-Zero/1 -> Demux1/1
  Demux1/1 -> Mux/1
  Demux1/2 -> Mux/2
  Demux1/3 -> Terminator/1
  Constant1/1 -> MatrixMultiply/1
  Demux/2 -> out_b1/1
  Demux/3 -> out_c1/1
  Demux/4 -> out_a2/1
  Demux/6 -> out_c2/1
  Demux/5 -> out_b2/1
  Demux/8 -> out_b3/1
  Demux/9 -> out_c3/1
  Demux/7 -> out_a3/1
